simulink model "PosControl_Sim"  (R2017b)
settings: Solver=ode4  StartTime=0.0  StopTime=2  FixedStep=0.001  RelTol=1e-3
InitFcn:
  | Init_control;
values from neighbouring files (symbols this model uses):
  DEG2RAD = 0.0174533    [Init_control.m]
  Kd_PITCH_AngleRate = 0.001    [Init_control.m]
  Kd_ROLL_AngleRate = 0.001    [Init_control.m]
  Kd_YAW_AngleRate = 0.00    (= 0)    [Init_control.m]
  Ki_PITCH_AngleRate = 0.02    [Init_control.m]
  Ki_ROLL_AngleRate = 0.02    [Init_control.m]
  Ki_YAW_AngleRate = 0.01    [Init_control.m]
  Kp_PITCH_ANGLE = 6.5    [Init_control.m]
  Kp_PITCH_AngleRate = 0.1    [Init_control.m]
  Kp_ROLL_ANGLE = 6.5    [Init_control.m]
  Kp_ROLL_AngleRate = 0.1    [Init_control.m]
  Kp_YAW_AngleRate = 0.5    [Init_control.m]
  Kpxp = 1.0    (= 1)    [Init_control.m]
  Kpyp = 1.0    (= 1)    [Init_control.m]
  Kpzp = 4.0    (= 4)    [Init_control.m]
  Kvxd = 0.01    [Init_control.m]
  Kvxi = 0.4    [Init_control.m]
  Kvxp = 2.5    [Init_control.m]
  Kvyd = 0.01    [Init_control.m]
  Kvyi = 0.4    [Init_control.m]
  Kvyp = 2.5    [Init_control.m]
  Kvzd = 0.005    [Init_control.m]
  Kvzi = 0.01    [Init_control.m]
  Kvzp = 0.45    [Init_control.m]
  MAX_CONTROL_ANGLE_PITCH = 35    [Init_control.m]
  MAX_CONTROL_ANGLE_RATE_PITCH = 220    [Init_control.m]
  MAX_CONTROL_ANGLE_RATE_ROLL = 220    [Init_control.m]
  MAX_CONTROL_ANGLE_RATE_Y = 200    [Init_control.m]
  MAX_CONTROL_ANGLE_ROLL = 35    [Init_control.m]
  MAX_CONTROL_VELOCITY_XY = 5    [Init_control.m]
  MAX_CONTROL_VELOCITY_Z = 3    [Init_control.m]
  ModelInit_AngEuler = [0, 0, 0]    [Init_control.m]
  ModelInit_PosE = [0, 0, -100]    [Init_control.m]
  ModelInit_Rads = 0    [Init_control.m]
  ModelInit_RateB = [0, 0, 0]    [Init_control.m]
  ModelInit_VelB = [0, 0, 0]    [Init_control.m]
  Saturation_I_ah = 3.43    [Init_control.m]
  Saturation_I_az = 5    [Init_control.m]
  Saturation_I_RP_Max = 0.3    [Init_control.m]
  Saturation_I_RP_Min = -0.3    [Init_control.m]
  Saturation_I_Y_Max = 0.2    [Init_control.m]
  Saturation_I_Y_Min = -0.2    [Init_control.m]
  THR_HOVER = 0.609    [Init_control.m]
undefined symbols (not defined in the file or in its folder): DiscIntNeverNeededParam, earthRadius, ModelParam_envGravityAcc, ModelParam_motorCr, ModelParam_motorJm, ModelParam_motorT, ModelParam_motorWb, ModelParam_rotorCm, ModelParam_rotorCt, ModelParam_uavCCm, ModelParam_uavCd, ModelParam_uavJ, ModelParam_uavMass, ModelParam_uavR, Receive, Send
libraries: simulink x8, aerolibfltsims x3, sharedutil x2, aerolibanimutils x1
(part 2 of 2)

== matlab function PosControl_Sim/Control System/InputConditioning1/deadzone4 ==
  data: u input; y output
function y = fcn(u)
%Function description:
%  Control the range of the remote control input from RCMin to RCMax, and
%  set a dead zone with a dead zone size of ±deadZone. The output y is
%  normalized to 0~1.You can get the RC calibration parameters in QGC.
RCMin = 1100;
RCMax = 1900;
RCMid = (RCMin + RCMax)/2;
deadZoneRate = 0.05;
deadZone = deadZoneRate*(RCMax - RCMin);
k = 1/(RCMax - RCMid - deadZone);
% saturation
if(u < RCMin)
    u = RCMin;
elseif(u > RCMax)
    u = RCMax;
end
% dead zone and normalize
 if(u > RCMid + deadZone)
    y = (u-RCMid - deadZone)*k;
 elseif(u < RCMid - deadZone)
     y = (u - RCMid + deadZone)*k;
 else
     y = 0;
 end

 end

== matlab function PosControl_Sim/Quadcopter Dynamics/Control Effectiveness Model/Propeller Model ==
  data: w input; R input; Fp output; Fd output; Mp output; Cm input; Ct input; Vb input; Cd input; wb input; Md output; Cdm input; Jrp input; Ga output
function [Fp, Fd, Mp, Md, Ga] = fcn(w, R, Cm, Ct, Vb, Cd,wb, Cdm, Jrp)
 %Function description:
 %  Obtain the force and torque acting on the body. The airframe of the
 %  quadrotor is as follows:
 %3↓   1↑
 %  \ /
 %  / \
 %2↑   4↓
 %↑ stands for counterclockwise and ↓stands for clockwise.
 %Input：
 %  w: motor speed，unit：rad/s
 %  R: body radius(m)
 %  Cm: torque coefficient
 %  Ct: thrust coefficient
 %  Vb: aircraft speed in the body coordinate system
 %  Cd: damping coefficient
 %  wb: angular velocity in the body coordinate system
 %  Cdm: damping moment coefficient vector
 %  Jrp:  moment of inertia of motor rotor + propeller
 %Output:
 %  Fp: thrust under the body coordinate system
 %  Fd: aerodynamic force under the body coordinate system
 %  Mp: torque under the body coordinate system
 %  Md: aerodynamic moment
 %  Ga: gyro moment
 M_rctcm = [-sin(pi/4)*R*Ct, sin(pi/4)*R*Ct, sin(pi/4)*R*Ct, -sin(pi/4)*R*Ct;
            sin(pi/4)*R*Ct, -sin(pi/4)*R*Ct, sin(pi/4)*R*Ct, -sin(pi/4)*R*Ct;
            Cm, Cm, -Cm, -Cm];
 Mp = M_rctcm*(w.^2);  % torque
 
 Fp = [0; 0; -sum(Ct*(w.^2))];  % thrust
 Fd = -Cd*Vb.*abs(Vb)*0.5;  % aerodynamic force
 Md = -Cdm.*wb.*abs(wb);  % aerodynamic moment
 % gyro moment
 Ga = zeros(3,1);
 Ga(1) = Jrp*wb(2)*( w(1) + w(2) - w(3) - w(4));
 Ga(2) = Jrp*wb(1)*(-w(1) - w(2) + w(3) + w(4));
end

== matlab function PosControl_Sim/Quadcopter Dynamics/Rigid Model/Rigid-Body Kinematic Model /Euler angle to quaternion ==
  data: EulerAngle input; q output
function q = fcn(EulerAngle)
%Function description:
%  Get quaternions from Euler angle
q0 =  cos(EulerAngle(1)/2)*cos(EulerAngle(2)/2)*cos(EulerAngle(3)/2) + sin(EulerAngle(1)/2)*sin((EulerAngle(2)/2))*sin((EulerAngle(3)/2));
q1 = sin(EulerAngle(1)/2)*cos(EulerAngle(2)/2)*cos(EulerAngle(3)/2) - cos(EulerAngle(1)/2)*sin((EulerAngle(2)/2))*sin((EulerAngle(3)/2));
q2 = cos(EulerAngle(1)/2)*sin(EulerAngle(2)/2)*cos(EulerAngle(3)/2) + sin(EulerAngle(1)/2)*cos((EulerAngle(2)/2))*sin((EulerAngle(3)/2));
q3 = cos(EulerAngle(1)/2)*cos(EulerAngle(2)/2)*sin(EulerAngle(3)/2) - sin(EulerAngle(1)/2)*sin((EulerAngle(2)/2))*cos((EulerAngle(3)/2));
q = [q0 q1 q2 q3]';

== matlab function PosControl_Sim/Control System/Subsystem/pwm_out2 ==
  data: Roll input; M1 output; Pitch input; Yaw input; Thrust input; M2 output; M3 output; M4 output
function [M1, M2, M3, M4] = motor_mixer(Roll, Pitch, Yaw, Thrust)
%Function description:
%  Control allocation. The quadrotor type is X-configuration,
%  and the airframe is as follows:
%3↓   1↑
 %  \ /
 %  / \
 %2↑   4↓
%Input：
%  Roll, Pitch, Yaw: attitude controller output.
%  Thrust

idle_PWM = 1000;
scale = 1000;

M1 = (Thrust - Roll + Pitch + Yaw) * scale + idle_PWM;
M2 = (Thrust + Roll - Pitch + Yaw) * scale + idle_PWM;
M3 = (Thrust + Roll + Pitch - Yaw) * scale + idle_PWM;
M4 = (Thrust - Roll - Pitch - Yaw) * scale + idle_PWM;

== matlab function PosControl_Sim/Quadcopter Dynamics/Rigid Model/Rigid-Body Kinematic Model /Quaternion to Euler ==
  data: q input; y output
function y = fcn(q)
 %Function description:
%  Quaternions to Euler
phi = atan2(2*(q(1)*q(2) + q(3)*q(4)), (1 - 2*(q(2)*q(2) + q(3)*q(3))));
theta = asin(2*(q(1)*q(3) - q(2)*q(4)));
psi = atan2(2*(q(1)*q(4) + q(2)*q(3)), (1 - 2*(q(3)*q(3) + q(4)*q(4))));
y = [phi theta psi];

== matlab function PosControl_Sim/Quadcopter Dynamics/Rigid Model/Rigid-Body Kinematic Model /Quaternion to rotation matrix ==
  data: q input; Reb output
function Reb = fcn(q)
%Function description;
%  The rotation matrix of the Aircraft-Body Coordinate Frame (ABCF) to the
%  Earth-Fixed Coordinate Frame (EFCF) is obtained from the quaternions
Reb = [q(1)*q(1) + q(2)*q(2) - q(3)*q(3) - q(4)*q(4), 2*(q(2)*q(3) - q(1)*q(4)), 2*(q(2)*q(4) + q(1)*q(3))
           2*(q(2)*q(3) + q(1)*q(4)), q(1)*q(1) - q(2)*q(2) + q(3)*q(3) - q(4)*q(4), 2*(q(3)*q(4) - q(1)*q(2))
           2*(q(2)*q(4) - q(1)*q(3)), 2*(q(3)*q(4) + q(1)*q(2)), q(1)*q(1) - q(2)*q(2) - q(3)*q(3) + q(4)*q(4)];

== matlab function PosControl_Sim/Quadcopter Dynamics/Rigid Model/Rigid-Body Kinematic Model /Quaternions model ==
  data: pqr input; qdot output; q input
function qdot = fcn(pqr, q)
%Function description:
%  Quaternions model
qdot = 0.5*[0, -pqr(1), -pqr(2), -pqr(3); pqr(1), 0, pqr(3), -pqr(2); pqr(2), -pqr(3), 0, pqr(1); pqr(3), pqr(2), -pqr(1), 0]*q;

== matlab function PosControl_Sim/Control System/InputConditioning1/f1 ==
  data: in input; y output; hover input
function y = thr_curve(in, hover)
%Function description:
%  throttle curve. When the throttle is in the middle position, the output
%  is hovering throttle value.
%Input:
%  in: normalized throttle, range from 0 to 1
%  hover: hovering throttle value
%Output:
%  y: processed throttle value
if in < 0.5
	y=2 * in * hover;
else
	y=hover + 2 * (in - 0.5) * (1.0 - hover);
end
